simulink model "pendule"  (R2017a)
settings: Solver=VariableStepAuto  StartTime=0.0  StopTime=10.0  RelTol=1e-3
undefined symbols (not defined in the file): g, l
libraries: simulink x1
settings Model: Creator=jky  LastModifiedBy=jky

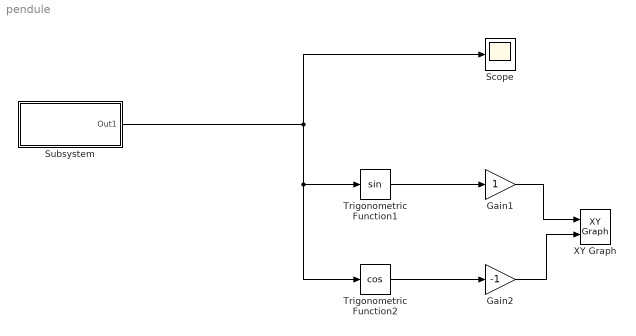
== system pendule ==
  Gain1 : Gain
  Gain2 : Gain  Gain=-1
  Scope : Scope
  Subsystem : Subsystem
  Trigonometric Function1 : Trigonometry
  Trigonometric Function2 : Trigonometry  Operator=cos
  XY Graph : simulink/Sinks/XY Graph  xmin=-1  xmax=1  ymin=-1  ymax=1  st=-1
  wires:
  Trigonometric Function1/1 -> Gain1/1
  Trigonometric Function2/1 -> Gain2/1
  Gain1/1 -> XY Graph/1
  Gain2/1 -> XY Graph/2
  Subsystem/1(Out1) -> Trigonometric Function1/1, Trigonometric Function2/1, Scope/1

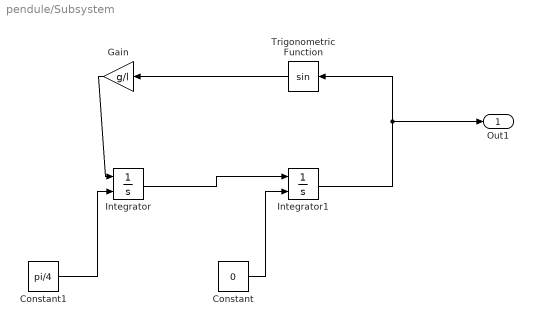
== system pendule/Subsystem ==
  Constant : Constant  Value=0
  Constant1 : Constant  Value=pi/4
  Gain : Gain  Gain=g/l
  Integrator : Integrator  InitialConditionSource=external
  Integrator1 : Integrator  InitialConditionSource=external
  Trigonometric Function : Trigonometry
  Out1 : Outport
  wires:
  Constant1/1 -> Integrator/2
  Integrator1/1 -> Out1/1, Trigonometric Function/1
  Trigonometric Function/1 -> Gain/1
  Gain/1 -> Integrator/1
  Integrator/1 -> Integrator1/1
  Constant/1 -> Integrator1/2
